simulink model "test"  (R2012b)
settings: Solver=ode45  StartTime=0.0  StopTime=10.0  RelTol=1e-3
settings Model: Creator=vesa  LastModifiedBy=vesa
settings OptimizationCC: InlineParams=on

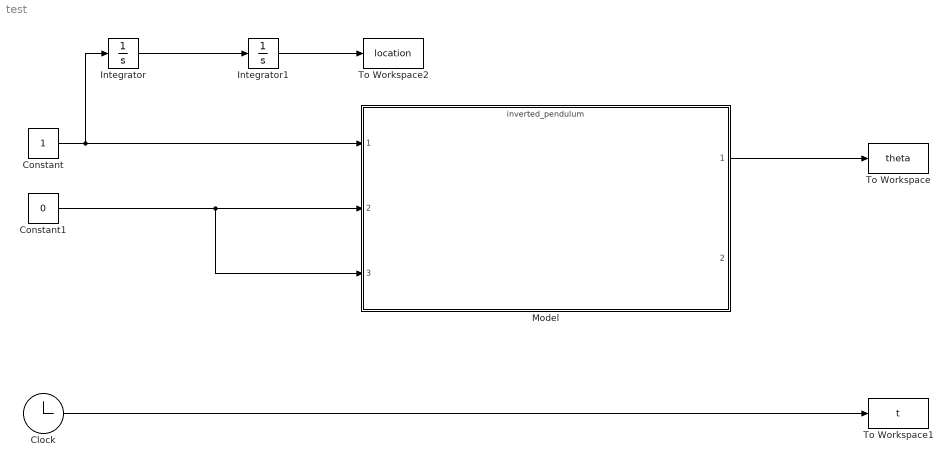
== system test ==
  Clock : Clock
  Constant : Constant
  Constant1 : Constant  Value=0
  Integrator : Integrator
  Integrator1 : Integrator
  Model : ModelReference  ModelNameDialog=inverted_pendulum  SimulationMode=Normal  ModelReferenceVersion=1.12  CopyOfModelName=inverted_pendulum  DefaultDataLogging=on
  To Workspace : ToWorkspace  VariableName=theta  SampleTime=-1
  To Workspace1 : ToWorkspace  VariableName=t  SampleTime=-1
  To Workspace2 : ToWorkspace  VariableName=location  SampleTime=-1
  wires:
  Constant/1 -> Integrator/1, Model/1
  Constant1/1 -> Model/3, Model/2
  Integrator/1 -> Integrator1/1
  Model/1 -> To Workspace/1
  Clock/1 -> To Workspace1/1
  Integrator1/1 -> To Workspace2/1
